simulink model "N1_SimpleDoublePipeHEX"  (R2020b)
settings: Solver=VariableStepAuto  StartTime=0.0  StopTime=10.0  RelTol=1e-3
settings Model: Creator=Rajas Gaikwad  LastModifiedBy=Rajas Gaikwad

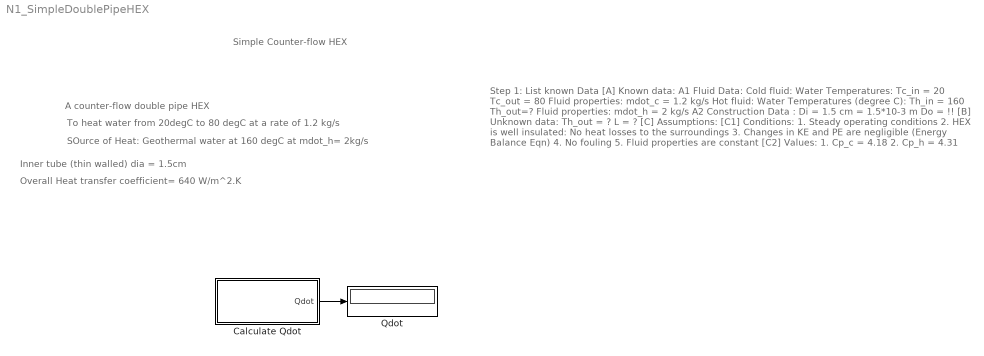
== system N1_SimpleDoublePipeHEX ==
  note: Step 1: List known Data
      |
      | [A] Known data:
      |
      | A1 Fluid Data:
      | Cold fluid: Water
      |
      | Temperatures:
      | Tc_in = 20
      | Tc_out = 80
      |
      | Fluid properties:
      | mdot_c = 1.2 kg/s
      |
      | Hot fluid: Water
      |
      | Temperatures (degree C):
      | Th_in = 160
      | Th_out=?
      |
      | Fluid properties:
      | mdot_h = 2 kg/s
      |
      | A2 Construction Data :
      |
      | Di = 1.5 cm = 1.5*10-3 m
      | Do = !!
      |
      | [B] Unknown data:
      |
      | Th_out = ?
      | L = ?
      |
      | [C] Assumptions:
      |
      | [C1] Conditions:
      | 1. Steady operating conditions
      | 2. HEX is well insulated: No heat losses to the surroundings
      | 3. Changes in KE and PE are negligible (Energy Balance Eqn)
      | 4. No fouling
      | 5. Fluid properties are constant
      |
      | [C2] Values:
      | 1. Cp_c = 4.18
      | 2. Cp_h = 4.31
  note: Overall Heat transfer coefficient= 640 W/m^2.K
  note: Inner tube (thin walled) dia = 1.5cm
  note: SOurce of Heat: Geothermal water at 160 degC at mdot_h= 2kg/s
  note: To heat water from 20degC to 80 degC at a rate of 1.2 kg/s
  note: A counter-flow double pipe HEX
  note: Simple Counter-flow HEX
  Calculate Qdot : Subsystem  mask{Th_in=160, Th_out=-999, Tc_in=20, Tc_out=80, mdot_h=2, mdot_c=1.2, Di=1.5, Cp_h=4.31, Cp_c=4.18}
      mask prompts: Th_in "Hot fluid inlet temperature (degree C)"; Th_out "Hot fluid outlet temperature (degree C)"; Tc_in "Cold fluid inlet temperature (degree C)"; Tc_out "Cold fluid outlet temperature (degree C)"; mdot_h "Hot fluid mass flow rate (kg/m^3)"; mdot_c "Cold fluid mass flow rate (kg/m^3)"; Di "Inside tube diameter (cm)"; Cp_h "Hot fluid specific heat (kJ/kg.K)"; Cp_c "Cold fluid specific heat (kJ/kg.K)"
      mask DialogControl Container4 Prompt: Fluid Data
      mask DialogControl Container6 Prompt: Temperatures
      mask DialogControl Container13 Prompt: Properties
      mask DialogControl Container14 Prompt: Design Data
      mask DialogControl Container9 Prompt: Assumed values
  Qdot : Display
  wires:
  Calculate Qdot/1(Qdot) -> Qdot/1

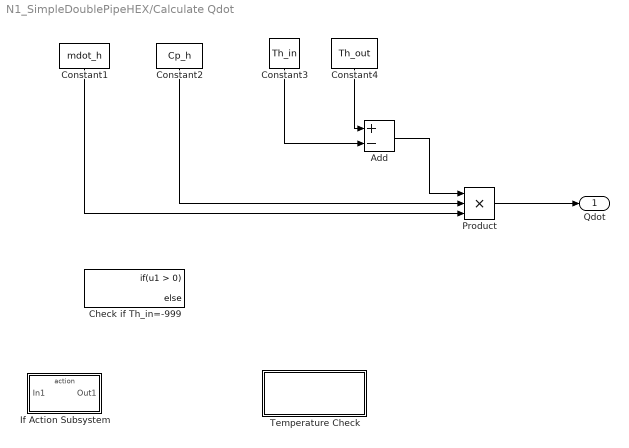
== system N1_SimpleDoublePipeHEX/Calculate Qdot ==
  Add : Sum  Inputs=+-
  Check if Th_in=-999 : If
  Constant1 : Constant  Value=mdot_h
  Constant2 : Constant  Value=Cp_h
  Constant3 : Constant  Value=Th_in
  Constant4 : Constant  Value=Th_out
  If Action Subsystem : Subsystem  TreatAsAtomicUnit=on
  Product : Product  Inputs=3
  "Temperature Check " : Subsystem
  Qdot : Outport
  wires:
  Product/1 -> Qdot/1
  Constant1/1 -> Product/3
  Constant2/1 -> Product/2
  Constant4/1 -> Add/1
  Constant3/1 -> Add/2
  Add/1 -> Product/1

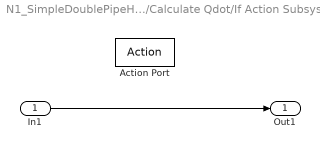
== system N1_SimpleDoublePipeHEX/Calculate Qdot/If Action Subsystem ==
  In1 : Inport
  Action Port : ActionPort
  Out1 : Outport
  wires:
  In1/1 -> Out1/1

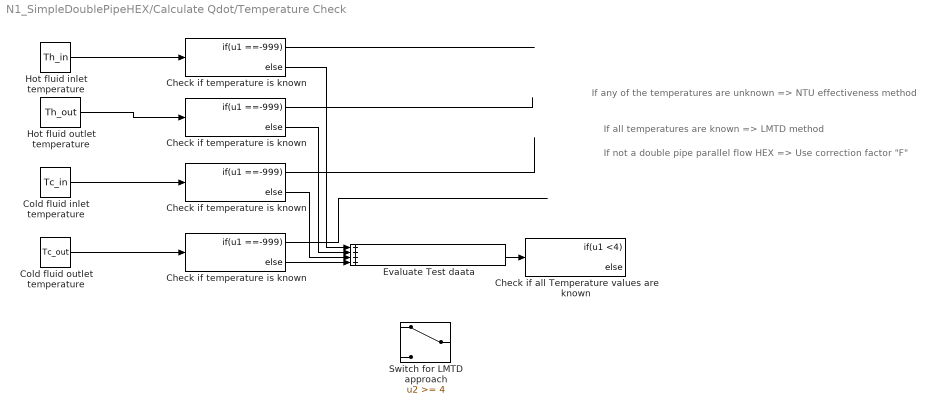
== system N1_SimpleDoublePipeHEX/Calculate Qdot/Temperature Check  ==
  note: If not a double pipe parallel flow HEX => Use correction factor "F"
  note: If all temperatures are known => LMTD method
  note: If any of the temperatures are unknown => NTU effectiveness method
  "   Check if temperature is known   " : If  IfExpression=u1 ==-999
  "  Check if all Temperature values are known  " : If  IfExpression=u1 <4
  "  Check if temperature is known  " : If  IfExpression=u1 ==-999
  " Check if temperature is known " : If  IfExpression=u1 ==-999
  Check if temperature is known : If  IfExpression=u1 ==-999
  Cold fluid inlet temperature : Constant  Value=Tc_in
  Cold fluid outlet temperature : Constant  Value=Tc_out
  Evaluate Test daata : Sum  Inputs=++++
  Hot fluid inlet temperature : Constant  Value=Th_in
  Hot fluid outlet temperature : Constant  Value=Th_out
  Switch for LMTD approach : Switch  Threshold=4
  wires:
  Hot fluid inlet temperature/1 -> Check if temperature is known/1
  Hot fluid outlet temperature/1 -> "  Check if temperature is known  "/1
  Cold fluid inlet temperature/1 -> " Check if temperature is known "/1
  Cold fluid outlet temperature/1 -> "   Check if temperature is known   "/1
  Check if temperature is known/2 -> Evaluate Test daata/1
  "  Check if temperature is known  "/2 -> Evaluate Test daata/2
  " Check if temperature is known "/2 -> Evaluate Test daata/3
  "   Check if temperature is known   "/2 -> Evaluate Test daata/4
  Evaluate Test daata/1 -> "  Check if all Temperature values are known  "/1
  Check if temperature is known/1 -> ?
  "  Check if temperature is known  "/1 -> ?
  " Check if temperature is known "/1 -> ?
  "   Check if temperature is known   "/1 -> ?
